simulink model "Vehicle_Model"  (R2018b)
settings: Solver=VariableStepAuto  StartTime=0.0  StopTime=60  FixedStep=0.00000000000000000000000000000000000000001  RelTol=1e-3
undefined symbols (not defined in the file or in its folder): Chassis8_Initial, Initial
(part 3 of 3)

== matlab function Vehicle_Model/MATLAB Function20 ==
  data: Fzo output; Ro output; q_Bz1 output; q_Bz2 output; q_Bz3 output; q_Bz4 output; q_Bz5 output; q_Bz9 output; q_Bz10 output; q_Cz1 output; q_Dz1 output; q_Dz2 output; q_Dz3 output; q_Dz4 output; q_Dz6 output; q_Dz7 output; q_Dz8 output; q_Dz9 output; q_Ez1 output; q_Ez2 output; q_Ez3 output; q_Ez4 output; q_Ez5 output; q_Hz1 output; q_Hz2 output; q_Hz3 output; q_Hz4 output; p_Cy1 output; p_Dy1 output; p_Dy2 output; p_Dy3 output; p_Ey1 output; p_Ey2 output; p_Ey3 output; p_Ey4 output; p_Ky1 output; p_Ky2 output; p_Ky3 output; p_Hy1 output; p_Hy2 output; p_Hy3 output; p_Vy1 output; p_Vy2 output; p_Vy3 output; p_Vy4 output; p_Cx1 output; p_Dx1 output; p_Dx2 output; p_Ex1 output; p_Ex2 output; p_Ex3 output; p_Ex4 output; p_Kx1 output; p_Kx2 output; p_Kx3 output; p_Hx1 output; p_Hx2 output; p_Vx1 output; p_Vx2 output
function [Fzo,Ro,q_Bz1,q_Bz2,q_Bz3,q_Bz4,q_Bz5,q_Bz9,q_Bz10,q_Cz1,q_Dz1,...
    q_Dz2,q_Dz3,q_Dz4,q_Dz6,q_Dz7,q_Dz8,q_Dz9,q_Ez1,q_Ez2,q_Ez3,q_Ez4,q_Ez5,...
    q_Hz1,q_Hz2,q_Hz3,q_Hz4,p_Cy1,p_Dy1,p_Dy2,p_Dy3,p_Ey1,p_Ey2,p_Ey3,...
    p_Ey4,p_Ky1,p_Ky2,p_Ky3,p_Hy1,p_Hy2,p_Hy3,p_Vy1,p_Vy2,p_Vy3,p_Vy4,...
    p_Cx1,p_Dx1,p_Dx2,p_Ex1,p_Ex2,p_Ex3,p_Ex4,p_Kx1,p_Kx2,p_Kx3,p_Hx1,...
    p_Hx2,p_Vx1,p_Vx2] = Hoosier_43131
% pacejka model coefficients provided by Stackpole Engineering Services
% for Hoosier tyre model 43131
% as found in the document 'SES_FSAE_Tiredata_Rev1'
% Specs:
% Size	20.0x6.0-13
% Pressure 12 psi


Fzo = 1114.01; % N
Ro = 0.25400; % m

% [ALIGNING COEFFICIENTS]
q_Bz1 =	7.31661;
q_Bz2 =	-1.88850;
q_Bz3 =	-1.22507;
q_Bz4 =	-8.00843;
q_Bz5 =	8.07362;
q_Bz9 =	0;
q_Bz10 = 0;
q_Cz1 =	1.24284;
q_Dz1 =	0.14936;
q_Dz2 =	-0.03781;
q_Dz3 =	0.64550;
q_Dz4 =	0.05268;
q_Dz6 =	-0.02434;
q_Dz7 =	0.01708;
q_Dz8 =	-1.08356;
q_Dz9 =	-0.40710;
q_Ez1 =	-3.38121;
q_Ez2 =	0.10261;
q_Ez3 =	-0.94450;
q_Ez4 =	0.36774;
q_Ez5 =	3.30689;
q_Hz1 =	-0.00061;
q_Hz2 =	-0.00550;
q_Hz3 =	0.38752;
q_Hz4 =	0.43969;

%  [LATERAL COEFFICIENTS]
p_Cy1 =	1.80000;
p_Dy1 =	2.45700;
p_Dy2 =	-0.59060;
p_Dy3 =	11.58940;
p_Ey1 =	0.97472;
p_Ey2 =	0.04076;
p_Ey3 =	0.11095;
p_Ey4 =	-1.20038;
p_Ky1 =	-37.72991;
p_Ky2 =	-1.22482;
p_Ky3 =	1.90662;
p_Hy1 =	0.00081;
p_Hy2 =	-0.00938;
p_Hy3 =	-0.12520;
p_Vy1 =	-0.01307;
p_Vy2 =	0.00121;
p_Vy3 =	-0.21872;
p_Vy4 =	1.77405;

% [LONGITUDINAL COEFFICIENTS]
p_Cx1 =  1.50000;
p_Dx1 =	2.22960;
p_Dx2 =	-0.26506;
p_Ex1 =	0.34731;
p_Ex2 =	-0.36673;
p_Ex3 =	-0.28130;
p_Ex4 =	-0.05543;
p_Kx1 =	46.06520;
p_Kx2 =	-29.43060;
p_Kx3 =	-0.45644;
p_Hx1 =	-0.00087;
p_Hx2 =	-0.00179;
p_Vx1 =	0.00295;
p_Vx2 =	-0.04174;


% export coefficients in structure for ease of passing between functions
% varList = who;
% initialiste oup_ut structure
% pacejka_coefs = struct;

% add all existing variables to struture
% for index = 1:numel(varList)
%     pacejka_coefs.(varList{index}) = eval(varList{index});
% end

== matlab function Vehicle_Model/Subsystem1/MATLAB Function8 ==
  data: Fz input; Fxo output; kappa input; alpha input; gam input; Fzo input; Ro input; q_Bz1 input; q_Bz2 input; q_Bz3 input; q_Bz4 input; q_Bz5 input; q_Bz9 input; q_Bz10 input; q_Cz1 input; q_Dz1 input; q_Dz2 input; q_Dz3 input; q_Dz4 input; q_Dz6 input; q_Dz7 input; q_Dz8 input; q_Dz9 input; q_Ez1 input; q_Ez2 input; q_Ez3 input; q_Ez4 input; q_Ez5 input; q_Hz1 input; q_Hz2 input; q_Hz3 input; q_Hz4 input; p_Cy1 input; p_Dy1 input; p_Dy2 input; p_Dy3 input; p_Ey1 input; p_Ey2 input; p_Ey3 input; p_Ey4 input; p_Ky1 input; p_Ky2 input; p_Ky3 input; p_Hy1 input; p_Hy2 input; p_Hy3 input; p_Vy1 input; p_Vy2 input; p_Vy3 input; p_Vy4 input; p_Cx1 input; p_Dx1 input; p_Dx2 input; p_Ex1 input; p_Ex2 input; p_Ex3 input; p_Ex4 input; p_Kx1 input; p_Kx2 input; p_Kx3 input; p_Hx1 input; p_Hx2 input; p_Vx1 input; p_Vx2 input; car_mu_scaling input; run_info input; Fyo output; Mzo output
function [Fxo,Fyo,Mzo] = Pacejka_Tyre_Model(Fz,kappa,alpha,gam,Fzo,Ro,...
    q_Bz1,q_Bz2,q_Bz3,q_Bz4,q_Bz5,q_Bz9,q_Bz10,q_Cz1,q_Dz1,...
    q_Dz2,q_Dz3,q_Dz4,q_Dz6,q_Dz7,q_Dz8,q_Dz9,q_Ez1,q_Ez2,q_Ez3,q_Ez4,q_Ez5,...
    q_Hz1,q_Hz2,q_Hz3,q_Hz4,p_Cy1,p_Dy1,p_Dy2,p_Dy3,p_Ey1,p_Ey2,p_Ey3,...
    p_Ey4,p_Ky1,p_Ky2,p_Ky3,p_Hy1,p_Hy2,p_Hy3,p_Vy1,p_Vy2,p_Vy3,p_Vy4,...
    p_Cx1,p_Dx1,p_Dx2,p_Ex1,p_Ex2,p_Ex3,p_Ex4,p_Kx1,p_Kx2,p_Kx3,p_Hx1,...
    p_Hx2,p_Vx1,p_Vx2,car_mu_scaling,run_info)
% Pacejka '96 tyre model
%
% Inputs:
% Fz:       normal force (N)
% kappa:    slip ratio (% between -1 and 1) +ve is driving, -ve is braking
% alpha:    slip angle (rad) +ve alpha generates +ve Fyo
% gam:      inclanation angle./camber (rad) +ve indicates top of tyre tipped
%           right
% Outputs:
% Fxo:      Longitudinal force (N)
% Fyo:      Lateral force (N)
% Mzo:      Aligning moment (Nm)


%% tyre coefficients
% each different type of tyre holds different scaling coefficients, load 
% these here. Also loaded are unloaded tyre radius and nominal wheel load

% unpack the structure holding the coefficients
% Get the field names of the structure.
% fields = fieldnames(pacejka_coefs, '-full');
% 
% for ii = 1:length(fields)
%     thisField = fields{ii};
%     create_variable = sprintf('%s = pacejka_coefs.%s;', thisField, thisField);
%     eval(create_variable);
% end
% clear('ii', 'thisField');
% clear('fields', 'create_variable');

%% register track conditions
% scaling factors affected by wet/dry conditions
% if strcmp(run_info.track_conditions,'dry')
    lambda_mux = 1; % peak friction coefficient
    lambda_muy = 1; % peak friction coefficient
% elseif strcmp(run_info.track_conditions,'wet')
%     lambda_mux = 0.5; % peak friction coefficient
%     lambda_muy = 0.5; % peak friction coefficient
% else
%     fprintf('Track conditions incorrectly specified: dry condtitions used \n');
%     lambda_mux = 1; % peak friction coefficient
%     lambda_muy = 1; % peak friction coefficient
% end

% modify with user scaling factor
lambda_mux = lambda_mux*car_mu_scaling;
lambda_muy = lambda_muy*car_mu_scaling;

%% scaling factors
% default values for these values is 1 (except lambda_muV=0)
lambda_Fzo = 1; % nominal rated load
lambda_muV = 0; % with slip speed Vx decaying friction
lambda_Kx = 1; % brake slip stiffness
lambda_Ky = 1; % cornering stiffness
lambda_Cx = 1; % shape factor
lambda_Cy = 1; % shape factor
lambda_Ex = 1; % curvature factor
lambda_Ey = 1; % curvature factor
lambda_Hx = 1; % horizontal shift
lambda_Hy = 1; % horizontal shift
lambda_Vx = 1; % vertical shift
lambda_Vy = 1; % vertical shift
lambda_Kygam = 1; % camber force stiffness
lambda_Kzgam = 1; % camber torque stiffness
lambda_t = 1; % pneumatic trail
lambda_Mr = 1; % residual torque
lambda_ygam = 1;

if ~isrow(kappa) || ~isrow(alpha) || ~isrow(gam)
    kappa = transpose(kappa);
    alpha = transpose(alpha);
    gam = transpose(gam);
end

% for ii=1:length(Fz)
%     %% derived inputs
     dfz = (Fz-Fzo)/Fzo; % normalised change in vertical load
    
    %% longitudinal force (pure longitudinal slip)
    S_Vx = Fz*(p_Vx1+p_Vx2.*dfz).*lambda_Vx.*lambda_mux;
    S_Hx = (p_Hx1+p_Hx2.*dfz).*lambda_Hx;
    kappa_x = kappa + S_Hx;
    K_xk = Fz*(p_Kx1+p_Kx2.*dfz).*exp(-p_Kx3.*dfz).*lambda_Kx;
    E_x = (p_Ex1+p_Ex2.*dfz+p_Ex3.*dfz.^2).*(1-p_Ex4.*sign(kappa_x)).*lambda_Ex;
    mu_x = (p_Dx1+p_Dx2.*dfz).*lambda_mux;
    D_x = mu_x.*Fz;
    C_x = p_Cx1.*lambda_Cx;
    B_x = K_xk./(C_x.*D_x);
    Fxo = D_x.*sin(C_x.*atan(B_x.*kappa_x - E_x.*(B_x.*kappa_x-atan(B_x.*kappa_x)))) + S_Vx;
    
    %% lateral force (pure lateral slip)
    gam_y = gam.*lambda_ygam;
    C_y = p_Cy1.*lambda_Cy;
    mu_y = (p_Dy1+p_Dy2.*dfz).*(1-p_Dy3.*gam.^2).*lambda_muy;
    D_y = mu_y.*Fz;
    S_Hy = (p_Hy1+p_Hy2.*dfz+p_Hy3.*gam).*lambda_Hy;
    alpha_y = alpha + S_Hy;
    E_y = (p_Ey1+p_Ey2.*dfz).*(1-(p_Ey3+p_Ey4.*gam_y).*sign(alpha_y)).*lambda_Ey;
    K_ya = p_Ky1.*Fzo.*sin(2.*atan(Fz./(p_Ky2.*Fzo.*lambda_Fzo))).*(1-p_Ky3.*abs(gam)).*lambda_Fzo.*lambda_Ky;
    B_y = K_ya./(C_y.*D_y);
    S_Vy = Fz.*((p_Vy1+p_Vy2.*dfz)+(p_Vy3+p_Vy4.*dfz).*gam.*lambda_Vy.*lambda_Kygam);
    Fyo = D_y.*sin(C_y.*atan(B_y.*alpha_y - E_y.*(B_y.*alpha_y-atan(B_y.*alpha_y)))) + S_Vy;
    
    %% aligning torque (pure side slip)
    B_t = (q_Bz1+q_Bz2.*dfz+q_Bz3.*dfz.^2).*(1+q_Bz4.*gam.*q_Bz5.*abs(gam)).*lambda_Ky./lambda_muy;
    C_t = q_Cz1;
    D_t = (q_Dz1+q_Dz2.*dfz).*(1+q_Dz3.*gam+q_Dz4.*gam.^2).*Ro.*lambda_t./Fzo;
    S_Ht = q_Hz1+q_Hz2.*dfz+(q_Hz3+q_Hz4.*dfz).*gam;
    alpha_t = alpha + S_Ht;
    E_t = (q_Ez1+q_Ez2.*dfz+q_Ez3.*dfz.^2).*(1+(q_Ez4+q_Ez5.*gam).*atan(B_t.*C_t.*alpha_t));
    B_r = (q_Bz9.*lambda_Ky./lambda_muy+q_Bz10.*B_y.*C_y);
    D_r = Fz.*((q_Dz6+q_Dz7.*dfz)+(q_Dz8+q_Dz9.*dfz).*gam).*Ro.*lambda_muy.*lambda_Mr;
    S_Hf = S_Hy + S_Vy./K_ya;
    alpha_r = alpha + S_Hf;
    Mzr = D_r.*cos(atan(B_r.*alpha_r)).*cos(alpha);
    t = D_t.*cos(C_t.*atan(B_t.*alpha_t-E_t.*(B_t.*alpha_t-atan(B_t.*alpha_t)))).*cos(alpha);
    Mzo = -t.*Fyo + Mzr;
    
% end

== matlab function Vehicle_Model/Subsystem1/MATLAB Function ==
  data: x input; F_z output; xdot input; k input; c input
function F_z = fcn(x,xdot,k,c)

F_z = k * x + c * xdot;

== matlab function Vehicle_Model/MATLAB Function21 ==
  data: whatever input; k_SFR output; Owen input; wants input; k_SFL output; k_SRR output; k_SRL output; c_SFR output; c_SFL output; c_SRR output; c_SRL output; k_TFR output; k_TFL output; k_TRR output; k_TRL output; c_TFR output; c_TFL output; c_TRR output; c_TRL output; k_RF output; k_RR output; k_FRIC output; c_RF output; c_RR output; c_FRIC output; gamma_FR output; gamma_FL output; gamma_RR output; gamma_RL output
function [k_SFR,k_SFL,k_SRR,k_SRL,c_SFR,c_SFL,c_SRR,c_SRL,k_TFR,k_TFL,...
    k_TRR,k_TRL,c_TFR,c_TFL,c_TRR,c_TRL,k_RF,k_RR,k_FRIC,c_RF,c_RR,...
    c_FRIC,gamma_FR,gamma_FL,gamma_RR,gamma_RL]...
    = Suspension_Mapping(whatever,Owen,wants)

% Suspension Stifnesses
k_SFR = 2000; %suspension stiffness front right (N/m)
k_SFL = 2000; %suspension stiffness front left (N/m)
k_SRR = 2000; %suspension stiffness rear right (N/m)
k_SRL = 2000; %suspension stiffness rear left (N/m)

% Tire Stifnesses
k_TFR = 15000; %tire stiffness front right (N/m)
k_TFL = 15000; %tire stiffness front left (N/m)
k_TRR = 15000; %tire stiffness rear right (N/m)
k_TRL = 15000; %tire stiffness rear left (N/m)

% Suspension Damping Coefficients
c_SFR = 1000; %suspension damping coefficient front right (Ns/m)
c_SFL = 1000; %suspension damping coefficient front left (Ns/m)
c_SRR = 1000; %suspension damping coefficientv rear right (Ns/m)
c_SRL = 1000; %suspension damping coefficient rear left (Ns/m)

% Tire Damping Coefficients
c_TFR = 500; %tire damping coefficient front right (Ns/m)
c_TFL = 500; %tire damping coefficient front left (Ns/m)
c_TRR = 500; %tire damping coefficientv rear right (Ns/m)
c_TRL = 500; %tire damping coefficient rear left (Ns/m)

% Roll Bar Stiffnesses
k_RF = 0; %front
k_RR = 0; %rear
k_FRIC = 0; %front to rear

% Roll Bar Damping
c_RF = 0; %front
c_RR = 0; %rear
c_FRIC = 0; %front to rear

% Camber (deg) (tilt right positive)
gamma_FRd = -2;
gamma_FLd = 2;
gamma_RRd = -1;
gamma_RLd = 1;

% Camber (Rad)
Deg2Rad = 0.0174533;
gamma_FR = gamma_FRd * Deg2Rad;
gamma_FL = gamma_FLd * Deg2Rad;
gamma_RR = gamma_RRd * Deg2Rad;
gamma_RL = gamma_RLd * Deg2Rad;

== matlab function Vehicle_Model/MATLAB Function22 ==
  data: g output
function g  = Environment_Parameters

g = 9.81;

== matlab function Vehicle_Model/Chassis Vertical 8DOF/MATLAB Function22 ==
  data: g input; F_zWFR output; m_WFR input; m_WFL input; m_WRR input; m_WRL input; F_zWFL output; F_zWRR output; F_zWRL output
function [F_zWFR,F_zWFL,F_zWRR,F_zWRL] = fcn(g,m_WFR,m_WFL,m_WRR,m_WRL)

F_zWFR = -g * m_WFR;
F_zWFL = -g * m_WFL;
F_zWRR = -g * m_WRR;
F_zWRL = -g * m_WRL;

== matlab function Vehicle_Model/MATLAB Function23 ==
  data: many input; ratio_FR output; angle_FR output; ratio_FL output; angle_FL output; ratio_RR output; angle_RR output; ratio_RL output; angle_RL output; to input; find input
function [ratio_FR,angle_FR,ratio_FL,angle_FL,ratio_RR,angle_RR,ratio_RL,...
    angle_RL] = Tyre_Slips(many,to,find)

ratio_FR = 0;
angle_FR = 0;
ratio_FL = 0;
angle_FL = 0;
ratio_RR = 0;
angle_RR = 0;
ratio_RL = 0;
angle_RL = 0;
